simulink subsystem "CTC_controller"  (R2023a)
settings: Solver=VariableStepAuto  StartTime=0.0  StopTime=10.0  RelTol=1e-3
libraries: robotcorelib x2, aerolibutil x2, dspinverses x1
settings Model: Creator=matte  LastModifiedBy=matte

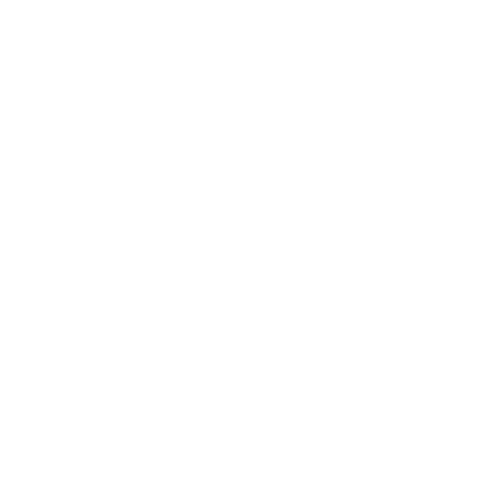
[thumbnail: Simulink's stored preview of the top-level diagram]
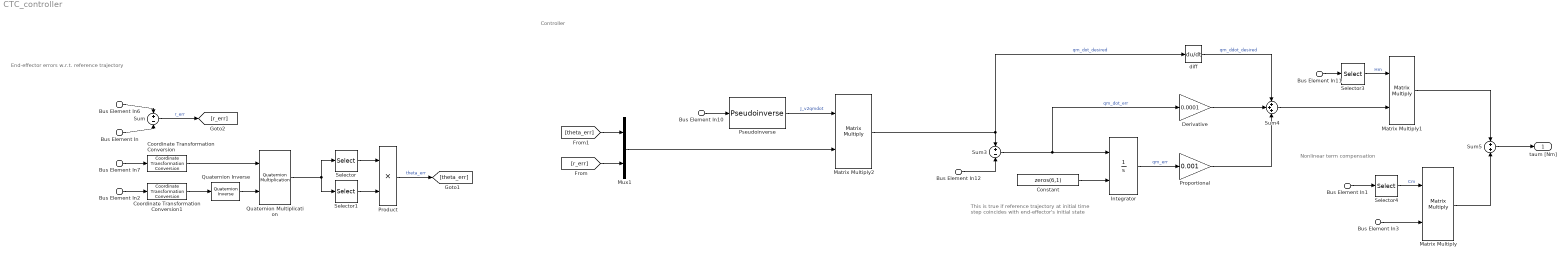
== system CTC_controller ==
  note: This is true if reference trajectory at initial time step coincides with end-effector's initial state
  note: Controller
  note: Nonlinear term compensation
  note: End-effector errors w.r.t. reference trajectory
  Bus Element In1 : Inport  PortName=robotState  Element=C
  Bus Element In3 : Inport  PortName=robotState  Element=qm_dot [rad/s]
  Bus Element In12 : Inport  PortName=robotState  Element=qm_dot [rad/s]
  Bus Element In6 : Inport  PortName=robotState  Element=eeState.p_ee [m]
  Bus Element In7 : Inport  PortName=robotState  Element=eeState.R_ee [rad]
  Bus Element In11 : Inport  PortName=robotState  Element=H
  Bus Element In10 : Inport  PortName=robotState  Element=J_qmdot2v
  Bus Element In : Inport  Port=2  PortName=referenceTrajectory  Element=p_ee
  Bus Element In2 : Inport  Port=2  PortName=referenceTrajectory  Element=R_ee
  Constant : Constant  Value=zeros(6,1)
  Coordinate Transformation Conversion : robotcorelib/Coordinate Transformation Conversion  InputRepresentation=Rotation Matrix  InputEulerSequence=ZYX  ShowTrVecInputPort=on  OutputRepresentation=Quaternion  OutputEulerSequence=ZYX  ShowTrVecOutputPort=on  SimulateUsing=Interpreted execution
      settings: LibrarySourceBlock=navlib/Utilities/Coordinate Transformation Conversion
  Coordinate Transformation Conversion1 : robotcorelib/Coordinate Transformation Conversion  InputRepresentation=Rotation Matrix  InputEulerSequence=ZYX  ShowTrVecInputPort=on  OutputRepresentation=Quaternion  OutputEulerSequence=ZYX  ShowTrVecOutputPort=on  SimulateUsing=Interpreted execution
      settings: LibrarySourceBlock=navlib/Utilities/Coordinate Transformation Conversion
  Derivative : Gain  Gain=0.0001
  Integrator : Integrator  InitialConditionSource=external  AbsoluteTolerance=opts.AbsTol
  Matrix Multiply : Product  Multiplication=Matrix(*)
  Matrix Multiply1 : Product  Multiplication=Matrix(*)
  Matrix Multiply2 : Product  Multiplication=Matrix(*)
  Mux1 : Mux  Inputs=2
  Product : Product
  Proportional : Gain  Gain=0.001
  Pseudoinverse : dspinverses/Pseudoinverse  wanterr=off  SimulateUsing=Interpreted execution
  Quaternion Inverse : aerolibutil/Quaternion Inverse
  Quaternion Multiplication : aerolibutil/Quaternion Multiplication
  Selector : Selector  InputPortWidth=4  IndexOptions=Index vector (dialog)  Indices=[1]  OutputSizes=1
  Selector1 : Selector  InputPortWidth=4  IndexOptions=Index vector (dialog)  Indices=[2:4]  OutputSizes=1
  Selector3 : Selector  NumberOfDimensions=2  InputPortWidth=3  IndexOptions=Index vector (dialog),Index vector (dialog)  Indices=7:12,7:12  OutputSizes=1,1
  Selector4 : Selector  NumberOfDimensions=2  InputPortWidth=3  IndexOptions=Index vector (dialog),Index vector (dialog)  Indices=7:12,7:12  OutputSizes=1,1
  Sum : Sum  Inputs=+-
  Sum3 : Sum  Inputs=+-
  Sum4 : Sum  Inputs=+++
  Sum5 : Sum
  diff : Derivative
  taum [Nm] : Outport
  wires:
  Bus Element In1/1 -> Selector4/1
  Bus Element In3/1 -> Matrix Multiply/2
  Bus Element In6/1 -> Sum/1
  Bus Element In/1 -> Sum/2
  Sum/1 -> [r_err]  "r_err"
  Bus Element In2/1 -> Coordinate Transformation Conversion1/1
  Bus Element In7/1 -> Coordinate Transformation Conversion/1
  Selector/1 -> Product/1
  Selector1/1 -> Product/2
  Quaternion Multiplication/1 -> Selector/1, Selector1/1
  Product/1 -> [theta_err]  "theta_err"
  [r_err] -> Mux1/2
  [theta_err] -> Mux1/1
  Bus Element In10/1 -> Pseudoinverse/1
  Matrix Multiply2/1 -> Sum3/1, diff/1  "qm_dot_desired"
  Bus Element In12/1 -> Sum3/2
  Bus Element In11/1 -> Selector3/1
  Mux1/1 -> Matrix Multiply2/2
  Coordinate Transformation Conversion1/1 -> Quaternion Inverse/1
  Quaternion Inverse/1 -> Quaternion Multiplication/2
  Coordinate Transformation Conversion/1 -> Quaternion Multiplication/1
  Selector3/1 -> Matrix Multiply1/1  "Hm"
  Selector4/1 -> Matrix Multiply/1  "Cm"
  Matrix Multiply/1 -> Sum5/2
  Pseudoinverse/1 -> Matrix Multiply2/1  "J_v2qmdot"
  Sum3/1 -> Integrator/1, Derivative/1  "qm_dot_err"
  diff/1 -> Sum4/1  "qm_ddot_desired"
  Integrator/1 -> Proportional/1  "qm_err"
  Constant/1 -> Integrator/2
  Derivative/1 -> Sum4/2
  Proportional/1 -> Sum4/3
  Sum4/1 -> Matrix Multiply1/2
  Matrix Multiply1/1 -> Sum5/1
  Sum5/1 -> taum [Nm]/1
